simulink model "Sampling"  (R2021a)
settings: Solver=VariableStepAuto  StartTime=0.0  StopTime=.01  RelTol=1e-3
settings Model: Creator=arabh  LastModifiedBy=arabh

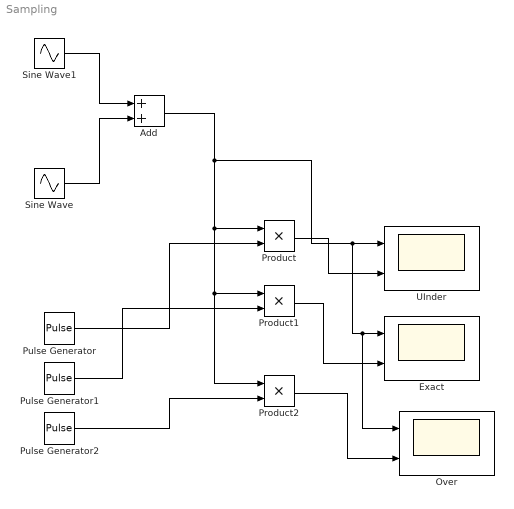
== system Sampling ==
  Add : Sum
  Exact : Scope  NumInputPorts=2
  "Over " : Scope  NumInputPorts=2
  Product : Product
  Product1 : Product
  Product2 : Product
  Pulse Generator : DiscretePulseGenerator  PulseType=Time based  Period=1/500  PulseWidth=25  VectorParams1D=off
  Pulse Generator1 : DiscretePulseGenerator  PulseType=Time based  Period=1/1000  PulseWidth=25  VectorParams1D=off
  Pulse Generator2 : DiscretePulseGenerator  PulseType=Time based  Period=1/1500  PulseWidth=25  VectorParams1D=off
  Sine Wave : Sin  Frequency=500  SampleTime=0  VectorParams1D=off
  Sine Wave1 : Sin  Frequency=500  SampleTime=0  VectorParams1D=off
  "UInder " : Scope  NumInputPorts=2
  wires:
  Pulse Generator/1 -> Product/2
  Sine Wave1/1 -> Add/1
  Sine Wave/1 -> Add/2
  Add/1 -> "Over "/1, Exact/1, "UInder "/1, Product2/1, Product1/1, Product/1
  Pulse Generator1/1 -> Product1/2
  Pulse Generator2/1 -> Product2/2
  Product/1 -> "UInder "/2
  Product1/1 -> Exact/2
  Product2/1 -> "Over "/2
